simulink model "nonlineardtm"  (R2018b)
settings: configuration reference "Physics" (kept outside this file)
model workspace (MAT data in the model file):
  MCOS : class17 (value not decoded)
undefined symbols (not defined in the file): Aerodynamics, Aligning, Antisway, Brakes, Compliance, ContactPatch, Environment, k1_TireFB_PT1, k1_WheelsFB_PT1, k2_TireFB_PT1, Kinematics, Lateral, Longitudinal, normalizeAngle, omega0_K_Vehicle_radps, omega0_Wheels_radps, Overturning, p_Tires_Pa, Rolling, Scaling, SensorData, Structural, TireSimulation, Turnslip, v0_K_Vehicle_mps, v0z_Wheels_mps, VehicleData, Vertical, Wheels, x0_verticaldynamics, z0_TireDeflection_m
libraries: vehdynlibtire x4, vehdynlibsuspension x2, vrlib x1, vehdynlibeom x1
(part 2 of 5)

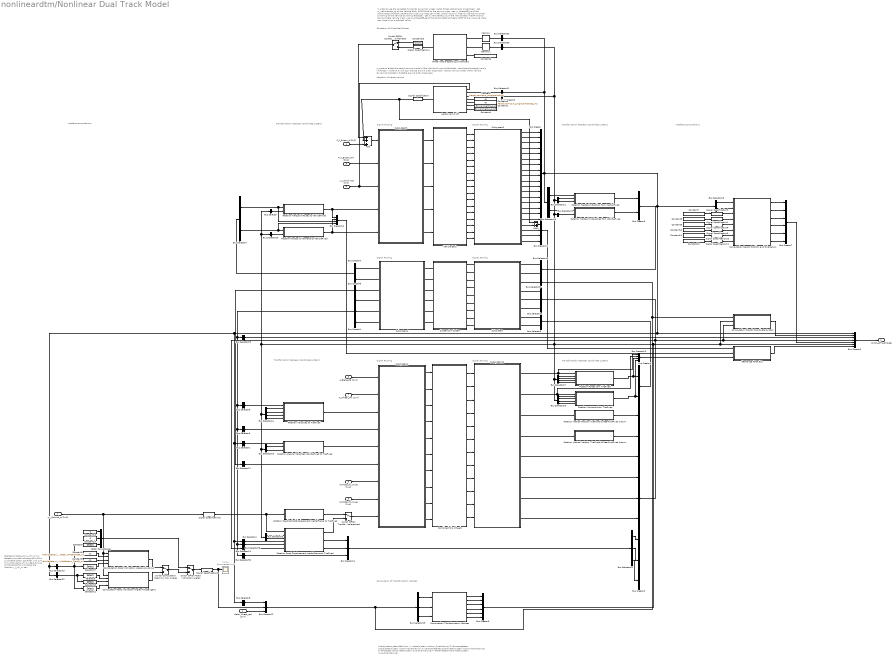
== system nonlineardtm/Nonlinear Dual Track Model ==
  note: Straßenkontaktpunkt  r_I_ITji_m zur Berechnung des Höhhenprofils führt zu algebraischen Schleifen und zum Simulationsabbruch
      | Zur Berechnung ds Höhenprofils wird daher die Position r_I_IAji_m der Anbindungspunkte an die Radaufhängungen verwendet
      | Alternative: Einführung von Verzögerungsgliedern oder Memory-Blöcken
  note: Koordinatensystemdefinition:
      | I: Inertialsystem (z-down Orientierung)
      | F: Fahrzeugfestes Koordinatensystem (z-down-Orientierung)
      | K: Karosseriefestes Koordinatensystem (z-down-Orientierung)
      | R: Radfestes Koordinatensystem (z-up-Orientierung)
      | T: Reifenfestes Koordinatensystem (z-up-Orientierung)
  note: Transformation
      | between coordinate systems
  note: Signal Routing
  note: Signal Routing
  note: Signal Routing
  note: Signal Routing
  note: Transformation
      | between coordinate systems
  note: Signal Routing
  note: Signal Routing
  note: Transformation
      | between coordinate systems
  note: Transformation
      | between coordinate systems
  note: Interface computations
  note: Interface Computations
  note: Computaion of Transformation Matrices
  note: Adaption of Aerodynamics
  note: In order to use the corrected horizontal dynamics wheel inertia forces according to d'Alembert:
      | - set m_VehicleMass_kg of the Vehicle Body 6DOF block to the sprung mass
      | - set m_WheelsFB_kg of the CombinedSlipWheels 2DOF to the unsprung mass per wheel (wheel mass)
      | In order to use the horizontal dynamics of the Vehicle Dynamics Blockset:
      | - set m_VehicleMass_kg of the Vehicle Body 6DOF block to the complete vehicle mass
      | - set m_WheelsFB_kg of the CombinedSlipWheels 2DOF to the unsprung mass per wheel or to a reduced value
  note: In order to adapt the aerodynamics model of the Vehicle Dynamics Blockset:
      | - calculate the aerodynamic lift forces in order to avoid sign change around pitch angle zero. Aerodynamics model of the Vehicle Dynamics blockset is bistable around pitch angle zero.
  note: Correction of d'Alembert Forces
  delta_Wheel_rad [1x4] : Inport
  T_Wheel_Nm [1x4] : Inport  Port=2
  p_Brake_Pa [1x4] : Inport  Port=3
  F_K_Extern_N [3x1] : Inport  Port=4
  T_K_Extern_Nm [3x1] : Inport  Port=5
  v_I_Wind_mps [3x1] : Inport  Port=6
  z_I_Ground_m [1x4] : Inport  Port=7
  lambda_Tji_muex [1x4] : Inport  Port=8
  lambda_Tji_muey [1x4] : Inport  Port=9
  Add : Sum  Inputs=+++
  Add1 : Sum  Inputs=-+
  Aerodynamic Lift : MATLAB Function  TreatAsAtomicUnit=on
  Bus Creator : BusCreator  Inputs=16
  Bus Creator1 : BusCreator  Inputs=3
  Bus Creator10 : BusCreator  Inputs=4
  Bus Creator11 : BusCreator  Inputs=5
  Bus Creator12 : BusCreator  Inputs=3
  Bus Creator13 : BusCreator  Inputs=4
  Bus Creator14 : BusCreator  Inputs=3
  Bus Creator2 : BusCreator  Inputs=9
  Bus Creator3 : BusCreator  Inputs=2
  Bus Creator4 : BusCreator  Inputs=2
  Bus Creator5 : BusCreator  Inputs=7
  Bus Creator6 : BusCreator  Inputs=2
  Bus Creator7 : BusCreator  Inputs=6
  Bus Creator8 : BusCreator  Inputs=1
  Bus Creator9 : BusCreator  Inputs=6
  Bus Selector{,12,20,33} (4 alike) : BusSelector  OutputSignals=A_K_F
  Bus Selector1 : BusSelector  OutputSignals=omega_K_IK_radps
  Bus Selector10 : BusSelector  OutputSignals=phi_IK_rad
  Bus Selector11 : BusSelector  OutputSignals=v_K_IK_mps
  Bus Selector13 : BusSelector  OutputSignals=r_I_IAji_m,v_K_IAji_mps
  Bus Selector14 : BusSelector  OutputSignals=h_ji_m
  Bus Selector15 : BusSelector  OutputSignals=re_ji_m
  Bus Selector16 : BusSelector  OutputSignals=r_F_IAji_m,v_F_IAji_mps
  Bus Selector17 : BusSelector  OutputSignals=F_F_Rji_N
  Bus Selector18 : BusSelector  OutputSignals=r_I_IK_m,A_K_I
  Bus Selector19 : BusSelector  OutputSignals=phi_IK_rad,chi_IO_rad,delta_ji_rad
  Bus Selector2 : BusSelector  OutputSignals=rz_F_Rji_m,re_ji_m,vz_F_Rji_m
  Bus Selector21 : BusSelector  OutputSignals=A_K_I,A_F_I
  Bus Selector22 : BusSelector  OutputSignals=r_I_IAji_m
  Bus Selector23 : BusSelector  OutputSignals=delta_ji_rad
  Bus Selector24 : BusSelector  OutputSignals=A_K_F,A_Rfl_F,A_Rfr_F,A_down_up
  Bus Selector25 : BusSelector  OutputSignals=A_K_F,A_down_up
  Bus Selector26 : BusSelector  OutputSignals=A_K_I,A_F_I
  Bus Selector27 : BusSelector  OutputSignals=A_K_F,A_Rfl_F,A_Rfr_F,A_down_up
  Bus Selector28 : BusSelector  OutputSignals=A_K_F,A_Rfl_F,A_Rfr_F,A_down_up
  Bus Selector29 : BusSelector  OutputSignals=h_ji_m,gamma-tau-nu_rad  OutputAsBus=on
  Bus Selector3 : BusSelector  OutputSignals=F_F_Tji_N,T_F_Tji_Nm
  Bus Selector30 : BusSelector  OutputSignals=v_F_IRji_mps
  Bus Selector31 : BusSelector  OutputSignals=r_I_IRji_m,r_I_ITji_m,v_F_IRji_mps
  Bus Selector32 : BusSelector  OutputSignals=a_K_IK_mps2
  Bus Selector4 : BusSelector  OutputSignals=r_I_IAji_m
  Bus Selector5 : BusSelector  OutputSignals=v_F_IRji_mps
  Bus Selector6 : BusSelector  OutputSignals=gamma-tau-nu_rad
  Bus Selector7 : BusSelector  OutputSignals=F_F_Aji_N,T_F_Aji_Nm
  Bus Selector8 : BusSelector  OutputSignals=phi_IK_rad
  Bus Selector9 : BusSelector  OutputSignals=A_K_I
  Combined Slip Wheels : Subsystem
  Computation Chassis Coordinate System : Subsystem
  Computation Road Inclination Angles Arkussinus : MATLAB Function  TreatAsAtomicUnit=on
  Computation Road Inclination Angles Arkustangens : MATLAB Function  TreatAsAtomicUnit=on
  Computation Sensor Position and Orientation : MATLAB Function  TreatAsAtomicUnit=on
  Computation Transformation Matrices : MATLAB Function  TreatAsAtomicUnit=on
  Constant : Constant  Value=Aerodynamics.cl_LongitudinalLift
  Constant1 : Constant  Value=Environment.t_Air_K
  Constant10 : Constant  Value=SensorData.phi0_K_KS1_rad
  Constant11 : Constant  Value=SensorData.phi0_K_KS2_rad
  Constant12 : Constant  Value=SensorData.phi0_K_KS3_rad
  Constant13 : Constant  Value=0
  Constant14 : Constant  Value=0
  Constant15 : Constant  Value=[0;0;0]
  Constant2 : Constant  Value=[VehicleData.l_WheelbaseF_m VehicleData.l_WheelbaseR_m]
  Constant3 : Constant  Value=Aerodynamics.A_LongitudinalDrag_m2
  Constant4 : Constant  Value=Environment.p_Air_Pa
  Constant5 : Constant  Value=[VehicleData.w_TrackF_m VehicleData.w_TrackR_m]
  Constant6 : Constant  Value=Wheels.m_WheelsFB_kg
  Constant7 : Constant  Value=SensorData.r_K_KS1_m
  Constant8 : Constant  Value=SensorData.r_K_KS2_m
  Constant9 : Constant  Value=SensorData.r_K_KS3_m
  Memory : Memory
  Memory1 : Memory
  Rearrange Force Bus : Subsystem
  Rotation Angular Velocities VehicleFixed to TireFixed : MATLAB Function  TreatAsAtomicUnit=on
  Rotation Forces from TireFixed : MATLAB Function  TreatAsAtomicUnit=on
  Rotation Hardpoint Forces to VehicleFixed : MATLAB Function  TreatAsAtomicUnit=on
  Rotation Hardpoint Moments to VehicleFixed : MATLAB Function  TreatAsAtomicUnit=on
  Rotation Hardpoint Position from InertialFixed : MATLAB Function  TreatAsAtomicUnit=on
  Rotation Hardpoint Velocities from VehicleFixed : MATLAB Function  TreatAsAtomicUnit=on
  Rotation Moments from TireFixed : MATLAB Function  TreatAsAtomicUnit=on
  Rotation Road Displacement InertialFrame to TireFixed : MATLAB Function  TreatAsAtomicUnit=on
  Rotation RoadVerticalDisplacement InertialFrame to TireFixed : Subsystem
  Rotation Velocities to TireFixed : MATLAB Function  TreatAsAtomicUnit=on
  Rotation Vertical Position TireFixed to RearAxleFixed z-down : Subsystem
  Rotation Vertical Velocity TireFixed to RearAxleFixed z-down : Subsystem
  Scope : Scope  Commented=on
  Selector20 : Selector  NumberOfDimensions=2  InputPortWidth=3  IndexOptions=Index vector (dialog),Select all  Indices=2,1  OutputSizes=1,1
  Selector21 : Selector  InputPortWidth=3  IndexOptions=Index vector (dialog)  Indices=3  OutputSizes=1
  Selector3 : Selector  InputPortWidth=3  IndexOptions=Index vector (dialog)  Indices=3  OutputSizes=1
  Selector37 : Selector  InputPortWidth=3  IndexOptions=Index vector (dialog)  Indices=3  OutputSizes=1
  Selector6 : Selector  NumberOfDimensions=2  InputPortWidth=3  IndexOptions=Index vector (dialog),Select all  Indices=1,1  OutputSizes=1,1
  Signal Specification{,1..4,8..11} (9 alike) : SignalSpecification  Dimensions=[3,1]
  Signal Specification5 : SignalSpecification  Dimensions=[1,4]
  Subsystem : Subsystem
  Subsystem1 : Subsystem
  Subsystem11 : Subsystem
  Subsystem2 : Subsystem
  Subsystem3 : Subsystem
  Subsystem4 : Subsystem
  Suspension System : Subsystem
  Switch Computation Road Inclination Angles : ManualSwitch
  Switch Off/On Correction Horizontal Dynamics Wheel Inertia according d'Alembert : ManualSwitch
  Switch Off/On Road Inclination Angles : ManualSwitch
  Switch Off/On Transformation Ground Displacement : ManualSwitch
  Vector Concatenate : Concatenate  NumInputs=3
  Vehicle Body : Subsystem
  Wheel Inertia according d'Alembert : MATLAB Function  TreatAsAtomicUnit=on
  SimDualTrackModel : Outport
  wires:
  Subsystem2/15(v_K_IAji_mps [3x4]) -> Bus Creator/15  "v_K_IAji_mps"
  Subsystem2/14(r_K_KAji_m [3x4]) -> Bus Creator/14  "r_K_KAji_m"
  Subsystem4/5(gamma-tau-nu_rad) -> Bus Creator1/2  "gamma-tau-nu_rad"
  Subsystem2/10(omega_K_IK_radps [3x1]) -> Bus Creator/10  "omega_K_IK_radps"
  Subsystem2/4(phi_IK_rad [3x1]) -> Bus Creator/4  "phi_IK_rad"
  v_I_Wind_mps [3x1]/1 -> Subsystem3/3(v_I_Wind_mps), Aerodynamic Lift/1(v_I_Wind_mps)  "v_I_Wind_mps"
  T_K_Extern_Nm [3x1]/1 -> Subsystem3/2(T_K_Extern_Nm)  "T_K_Ext_Nm"
  Add/1 -> Subsystem3/1(F_K_Extern_N)  "F_K_Ext_N"
  Subsystem11/6(omegay_Rji_Rji_radps) -> Bus Creator2/4  "omegay_Rji_Rji_radps"
  Subsystem11/4(vz_Tji_Rji_mps) -> Rotation Vertical Velocity TireFixed to RearAxleFixed z-down/1(vz_Tji_Rji_mps)  "vz_Tji_Rji_mps"
  Bus Creator2/1 -> Bus Selector15/1, Bus Selector2/1, Bus Creator5/4, Computation Chassis Coordinate System/3(Wheel)  "SimWheel"
  Bus Selector2/1 -> Subsystem/4(rz_F_IRji_m)  "<rz_F_Rji_m>"
  Bus Selector2/2 -> Subsystem/5(re_Rji_m)  "<re_ji_m>"
  Bus Selector2/3 -> Subsystem/6(vz_F_IRji_mps)  "<vz_F_Rji_m>"
  Bus Creator3/1 -> Bus Selector3/1
  Bus Selector3/1 -> Subsystem/7(F_F_Tji_N)  "<F_F_Tji_N>"
  Bus Selector3/2 -> Subsystem/8(T_F_Tji_Nm)  "<T_F_Tji_Nm>"
  z_I_Ground_m [1x4]/1 -> Signal Specification5/1, Computation Road Inclination Angles Arkustangens/1(z_I_Ground_m), Computation Road Inclination Angles Arkussinus/1(z_I_Ground_m)
  Subsystem2/1(r_I_IK_m [3x1]) -> Bus Creator/1  "r_I_IK_m"
  Subsystem2/2(v_I_IK_mps [3x1]) -> Bus Creator/2  "v_I_IK_mps"
  Subsystem2/13(v_I_IAji_mps [3x4]) -> Bus Creator/13  "v_I_IAji_mps"
  Subsystem2/7(v_K_IK_mps [3x1]) -> Bus Creator/7  "v_K_IK_mps"
  Subsystem2/8(a_K_IK_mps2 [3x1]) -> Bus Creator/8  "a_K_IK_mps2"
  Bus Selector8/1 -> Bus Creator12/1  "<phi_IK_rad>"
  Bus Selector1/1 -> Rotation Angular Velocities VehicleFixed to TireFixed/1(omega_K_IK_radps)  "<omega_K_IK_radps>"
  Bus Selector6/1 -> Subsystem1/4(gamma-tau-nu_rad)  "<gamma-tau-nu_rad>"
  Bus Creator4/1 -> Bus Selector7/1
  Bus Creator5/1 -> SimDualTrackModel/1
  Bus Creator1/1 -> Bus Selector30/1, Bus Selector14/1, Bus Selector6/1, Bus Selector5/1, Bus Selector29/1
  Subsystem2/16(A_K_I [3x3]) -> Bus Creator/16  "A_K_I"
  Subsystem2/12(r_I_IAji_m [3x4]) -> Bus Creator/12  "r_I_IAji_m"
  Subsystem11/5(re_ji_m) -> Bus Creator2/3  "re_ji_m"
  Bus Selector7/1 -> Bus Creator10/3, Rotation Hardpoint Forces to VehicleFixed/1(F_F_Aji_N)  "<F_F_Aji_N>"
  Bus Selector7/2 -> Bus Creator10/4, Rotation Hardpoint Moments to VehicleFixed/1(T_F_Aji_Nm)  "<T_F_Aji_Nm>"
  Rotation Hardpoint Position from InertialFixed/1(r_F_IAji_m) -> Bus Creator6/1  "r_F_IAji_m"
  Rotation Hardpoint Forces to VehicleFixed/1(F_K_Aji_N) -> Bus Creator10/1, Subsystem3/4(F_K_Aji_N)  "F_K_Aji_N"
  Rotation Hardpoint Moments to VehicleFixed/1(T_K_Aji_Nm) -> Bus Creator10/2, Subsystem3/5(T_K_Aji_Nm)  "T_K_Aji_Nm"
  Bus Selector5/1 -> Rotation Velocities to TireFixed/1(v_F_IRji_mps)  "<v_F_IRji_mps>"
  Rotation Velocities to TireFixed/1(v_Tji_Rji_mps) -> Subsystem1/3(v_Tji_Rji_mps)  "v_Tji_Rji_mps"
  Bus Selector10/1 -> Selector21/1, Selector37/1, Selector3/1  "<phi_IK_rad>"
  Constant2/1 -> Computation Road Inclination Angles Arkussinus/2(l_WheelbaseFB_m)
  Constant5/1 -> Computation Road Inclination Angles Arkussinus/3(w_TrackFB_m)
  Bus Selector13/2 -> Rotation Hardpoint Velocities from VehicleFixed/1(v_K_IAji_mps)  "<v_K_IAji_mps>"
  Signal Specification2/1 -> Bus Creator12/2, Scope/1  "chi_IO_rad"
  Bus Selector13/1 -> Rotation Hardpoint Position from InertialFixed/1(r_I_IAji_m)  "<r_I_IAji_m>"
  Bus Selector4/1 -> Rotation Road Displacement InertialFrame to TireFixed/4(r_I_IAji_m)  "<r_I_IAji_m>"
  Bus Selector14/1 -> Rotation Road Displacement InertialFrame to TireFixed/5(h_ji_m)  "<h_ji_m>"
  Bus Selector15/1 -> Rotation Road Displacement InertialFrame to TireFixed/6(re_ji_m)  "<re_ji_m>"
  Bus Selector16/1 -> Subsystem/1(r_F_IAji_m)  "<r_F_IAji_m>"
  Bus Selector16/2 -> Subsystem/2(v_F_IAji_mps)  "<v_F_IAji_mps>"
  Bus Creator6/1 -> Bus Selector16/1
  Subsystem11/7(kappa_ji) -> Bus Creator2/5  "kappa_ji"
  Subsystem11/8(alpha_ji_rad) -> Bus Creator2/6  "alpha_ji_rad"
  Rotation Road Displacement InertialFrame to TireFixed/3(r_I_ITji_m) -> Bus Creator14/2  "r_I_ITji_m"
  Bus Selector18/2 -> Computation Sensor Position and Orientation/2(A_K_I)  "<A_K_I>"
  Computation Sensor Position and Orientation/6(A_S3_I) -> Bus Creator7/6  "A_S3_I"
  Computation Sensor Position and Orientation/1(r_I_IS1_m) -> Bus Creator7/1  "r_I_IS1_m"
  Computation Sensor Position and Orientation/2(r_I_IS2_m) -> Bus Creator7/2  "r_I_IS2_m"
  Computation Sensor Position and Orientation/3(r_I_IS3_m) -> Bus Creator7/3  "r_I_IS3_m"
  Computation Sensor Position and Orientation/4(A_S1_I) -> Bus Creator7/4  "A_S1_I"
  Computation Sensor Position and Orientation/5(A_S2_I) -> Bus Creator7/5  "A_S2_I"
  Bus Creator7/1 -> Bus Creator5/5  "SimSensor"
  Bus Selector18/1 -> Computation Sensor Position and Orientation/1(r_I_IK_m)  "<r_I_IK_m>"
  Constant7/1 -> Signal Specification3/1
  Constant8/1 -> Signal Specification1/1
  Constant9/1 -> Signal Specification8/1
  Constant10/1 -> Signal Specification9/1
  Constant11/1 -> Signal Specification10/1
  Constant12/1 -> Signal Specification11/1
  Subsystem11/1(F_Tji_Tji_N) -> Rotation Forces from TireFixed/1(F_Tji_Tji_N), Bus Creator13/1  "F_Tji_Tji_N"
  Rotation Hardpoint Velocities from VehicleFixed/1(v_F_IAji_mps) -> Bus Creator6/2  "v_F_IAji_mps"
  Rotation Angular Velocities VehicleFixed to TireFixed/1(omega_Tji_ITji_radps) -> Subsystem1/5(omega_Tji_ITji_radps)  "omega_Tji_ITji_radps"
  Signal Specification5/1 -> Rotation RoadVerticalDisplacement InertialFrame to TireFixed/1(z_I_Ground_m), Rotation Road Displacement InertialFrame to TireFixed/1(z_I_Ground_m)
  Subsystem4/3(F_F_Rji_N) -> Bus Creator8/1  "F_F_Rji_N"
  delta_Wheel_rad [1x4]/1 -> Bus Creator12/3  "delta_ji_rad"
  Rotation Forces from TireFixed/1(F_F_Tji_N) -> Bus Creator13/3, Bus Creator3/1  "F_F_Tji_N"
  Rotation Moments from TireFixed/1(T_F_Tji_Nm) -> Bus Creator13/4, Bus Creator3/2  "T_F_Tji_Nm"
  Rotation Vertical Position TireFixed to RearAxleFixed z-down/1(rz_F_Rji_m) -> Bus Creator2/1  "rz_F_Rji_m"
  Rotation Vertical Velocity TireFixed to RearAxleFixed z-down/1(vz_F_Rji_mps) -> Bus Creator2/2  "vz_F_Rji_m"
  Subsystem/1(VehP [3x4]) -> Suspension System/1(VehP [3x4])
  Subsystem/2(VehV [3x4]) -> Suspension System/2(VehV [3x4])
  Subsystem/3(StrgAngF [1x2]) -> Suspension System/3(StrgAngF [1x2])
  Subsystem/4(WhlPz [1x4]) -> Suspension System/4(WhlPz [1x4])
  Subsystem/5(WhlRe [1x4]) -> Suspension System/5(WhlRe [1x4])
  Subsystem/6(WhlVz [1x4]) -> Suspension System/6(WhlVz [1x4])
  Subsystem/7(WhlFx [1x4]) -> Suspension System/7(WhlFx [1x4])
  Subsystem/8(WhlFy [1x4]) -> Suspension System/8(WhlFy [1x4])
  Subsystem/9(WhlM [3x4]) -> Suspension System/9(WhlM [3x4])
  Suspension System/1(VehF [3x4]) -> Subsystem4/1(VehF [3x4])
  Suspension System/2(VehM [3x4]) -> Subsystem4/2(VehM [3x4])
  Suspension System/3(WhlF [3x4]) -> Subsystem4/3(WhlF [3x4])
  Suspension System/4(WhlV [3x4]) -> Subsystem4/4(WhlV [3x4])
  Suspension System/5(WhlAng [3x4]) -> Subsystem4/5(WhlAng [3x4])
  Suspension System/6(SuspH [1x4]) -> Subsystem4/6(SuspH [1x4])
  Subsystem4/1(F_F_Aji_N) -> Bus Creator4/1  "F_F_Aji_N"
  Subsystem4/2(T_F_Aji_Nm) -> Bus Creator4/2  "T_F_Aji_Nm"
  Subsystem4/6(h_ji_m) -> Bus Creator1/3  "h_ji_m"
  Subsystem4/4(v_F_IRji_mps) -> Bus Creator1/1  "v_F_IRji_mps"
  Constant13/1 -> Vector Concatenate/1
  Constant14/1 -> Vector Concatenate/2
  Selector3/1 -> Vector Concatenate/3
  Selector37/1 -> Computation Road Inclination Angles Arkussinus/4(phiz_IK_rad)
  Vector Concatenate/1 -> Switch Off/On Road Inclination Angles/1
  Selector6/1 -> Computation Road Inclination Angles Arkustangens/2(rx_I_IAji_m)
  Selector20/1 -> Computation Road Inclination Angles Arkustangens/3(ry_I_IAji_m)
  Selector21/1 -> Computation Road Inclination Angles Arkustangens/4(phiz_IK_rad)
  Computation Road Inclination Angles Arkussinus/1(chi) -> Switch Computation Road Inclination Angles/1
  Computation Road Inclination Angles Arkustangens/1(chi) -> Switch Computation Road Inclination Angles/2
  Signal Specification3/1 -> Computation Sensor Position and Orientation/3(r_K_KS1_m)
  Signal Specification1/1 -> Computation Sensor Position and Orientation/4(r_K_KS2_m)
  Signal Specification8/1 -> Computation Sensor Position and Orientation/5(r_K_KS3_m)
  Signal Specification9/1 -> Computation Sensor Position and Orientation/6(phi0_K_KS1_rad)
  Signal Specification10/1 -> Computation Sensor Position and Orientation/7(phi0_K_KS2_rad)
  Signal Specification11/1 -> Computation Sensor Position and Orientation/8(phi0_K_KS3_rad)
  Subsystem2/9(vdot_K_IK_mps2 [3x1]) -> Bus Creator/9  "vdot_K_IK_mps2"
  Subsystem3/5(MSusp [3x4]) -> Vehicle Body/5(MSusp [3x4])
  Combined Slip Wheels/1(Fx [1x4]) -> Subsystem11/1(Fx [1x4])
  Combined Slip Wheels/2(Fy [1x4]) -> Subsystem11/2(Fy [1x4])
  Combined Slip Wheels/3(Fz [1x4]) -> Subsystem11/3(Fz [1x4])
  Combined Slip Wheels/5(My [1x4]) -> Subsystem11/5(My [1x4])
  Combined Slip Wheels/6(Mz [1x4]) -> Subsystem11/6(Mz [1x4])
  Combined Slip Wheels/7(z [1x4]) -> Subsystem11/7(z [1x4])
  Combined Slip Wheels/8(zdot [1x4]) -> Subsystem11/8(zdot [1x4])
  Combined Slip Wheels/9(Re [1x4]) -> Subsystem11/9(Re [1x4])
  Combined Slip Wheels/10(omega [1x4]) -> Subsystem11/10(omega [1x4])
  Combined Slip Wheels/11(Kappa [1x4]) -> Subsystem11/11(Kappa [1x4])
  Subsystem11/2(T_Tji_Tji_Nm) -> Rotation Moments from TireFixed/1(T_Tji_Tji_Nm), Bus Creator13/2  "T_Tji_Tji_Nm"
  Subsystem11/3(rz_Tji_Rji_m) -> Rotation Vertical Position TireFixed to RearAxleFixed z-down/1(rz_Tji_Rji_m)  "rz_Tji_Rji_m"
  p_Brake_Pa [1x4]/1 -> Subsystem1/1(p_Brake_Pa)
  T_Wheel_Nm [1x4]/1 -> Subsystem1/2(T_Wheel_Nm)
  lambda_Tji_muex [1x4]/1 -> Subsystem1/7(lambda_Tji_muex [1x4])
  lambda_Tji_muey [1x4]/1 -> Subsystem1/8(lambda_Tji_muey [1x4])
  Switch Off/On Transformation Ground Displacement/1 -> Subsystem1/9(z_Tji_Ground_m [1x4])
  Rotation RoadVerticalDisplacement InertialFrame to TireFixed/1(z_Tji_Ground_m) -> Switch Off/On Transformation Ground Displacement/1  "z_Tji_Ground_m"
  Rotation Road Displacement InertialFrame to TireFixed/1(z_Tji_Ground_m) -> Switch Off/On Transformation Ground Displacement/2  "z_Tji_Ground_m"
  Bus Creator8/1 -> Bus Selector17/1
  Bus Selector17/1 -> Subsystem1/6(F_F_Rji_N [3x4])  "<F_F_Rji_N>"
  Switch Computation Road Inclination Angles/1 -> Switch Off/On Road Inclination Angles/2
  Switch Off/On Road Inclination Angles/1 -> Signal Specification2/1
  Subsystem1/1(BrkPrs [1x4]) -> Combined Slip Wheels/1(BrkPrs [1x4])
  Subsystem1/2(AxlTrq [1x4]) -> Combined Slip Wheels/2(AxlTrq [1x4])
  Subsystem1/3(Vx [1x4]) -> Combined Slip Wheels/3(Vx [1x4])
  Subsystem1/4(Vy [1x4]) -> Combined Slip Wheels/4(Vy [1x4])
  Subsystem1/5(Camber [1x4]) -> Combined Slip Wheels/5(Camber [1x4])
  Subsystem1/6(YawRate [1x4]) -> Combined Slip Wheels/6(YawRate [1x4])
  Subsystem1/7(Prs [1x4]) -> Combined Slip Wheels/7(Prs [1x4])
  Subsystem1/8(Gnd [1x4]) -> Combined Slip Wheels/8(Gnd [1x4])
  Subsystem1/9(Fext [1x4]) -> Combined Slip Wheels/9(Fext [1x4])
  Subsystem1/10(ScaleFctrs [27x4]) -> Combined Slip Wheels/10(ScaleFctrs [27x4])
  Combined Slip Wheels/12(Alpha [1x4]) -> Subsystem11/12(Alpha [1x4])
  Computation Transformation Matrices/1(A_K_I) -> Bus Creator9/1  "A_K_I"
  Computation Transformation Matrices/2(A_K_F) -> Bus Creator9/2  "A_K_F"
  Computation Transformation Matrices/3(A_F_I) -> Bus Creator9/3  "A_F_I"
  Computation Transformation Matrices/4(A_Rfl_F) -> Bus Creator9/4  "A_Rfl_F"
  Computation Transformation Matrices/5(A_Rfr_F) -> Bus Creator9/5  "A_Rfr_F"
  Computation Transformation Matrices/6(A_down_up) -> Bus Creator9/6  "A_down_up"
  Bus Selector/1 -> Rotation Hardpoint Forces to VehicleFixed/2(A_K_F)  "<A_K_F>"
  Bus Selector20/1 -> Rotation Hardpoint Moments to VehicleFixed/2(A_K_F)  "<A_K_F>"
  Bus Selector12/1 -> Rotation Hardpoint Velocities from VehicleFixed/2(A_K_F)  "<A_K_F>"
  Bus Selector21/1 -> Rotation Hardpoint Position from InertialFixed/2(A_K_I)  "<A_K_I>"
  Bus Selector21/2 -> Rotation Hardpoint Position from InertialFixed/3(A_F_I)  "<A_F_I>"
  Bus Selector24/1 -> Rotation Velocities to TireFixed/2(A_K_F)  "<A_K_F>"
  Bus Selector24/2 -> Rotation Velocities to TireFixed/3(A_Rfl_F)  "<A_Rfl_F>"
  Bus Selector24/3 -> Rotation Velocities to TireFixed/4(A_Rfr_F)  "<A_Rfr_F>"
  Bus Selector24/4 -> Rotation Velocities to TireFixed/5(A_down_up)  "<A_down_up>"
  Bus Selector25/1 -> Rotation Angular Velocities VehicleFixed to TireFixed/2(A_K_F)  "<A_K_F>"
  Bus Selector25/2 -> Rotation Angular Velocities VehicleFixed to TireFixed/3(A_down_up)  "<A_down_up>"
  Bus Selector26/1 -> Rotation Road Displacement InertialFrame to TireFixed/2(A_K_I)  "<A_K_I>"
  Bus Selector26/2 -> Rotation Road Displacement InertialFrame to TireFixed/3(A_F_I)  "<A_F_I>"
  Bus Selector27/1 -> Rotation Forces from TireFixed/2(A_K_F)  "<A_K_F>"
  Bus Selector27/2 -> Rotation Forces from TireFixed/3(A_Rfl_F)  "<A_Rfl_F>"
  Bus Selector27/3 -> Rotation Forces from TireFixed/4(A_Rfr_F)  "<A_Rfr_F>"
  Bus Selector27/4 -> Rotation Forces from TireFixed/5(A_down_up)  "<A_down_up>"
  Bus Selector28/1 -> Rotation Moments from TireFixed/2(A_K_F)  "<A_K_F>"
  Bus Selector28/2 -> Rotation Moments from TireFixed/3(A_Rfl_F)  "<A_Rfl_F>"
  Bus Selector28/3 -> Rotation Moments from TireFixed/4(A_Rfr_F)  "<A_Rfr_F>"
  Bus Selector28/4 -> Rotation Moments from TireFixed/5(A_down_up)  "<A_down_up>"
  Bus Selector22/1 -> Selector20/1, Selector6/1  "<r_I_IAji_m>"
  Subsystem2/17(F_K_g_N [3x1]) -> Bus Creator11/1  "F_K_g_N"
  Add1/1 -> Bus Creator11/2  "F_K_d_N"
  Subsystem2/19(T_K_d_Nm [3x1]) -> Bus Creator11/3  "T_K_d_Nm"
  Subsystem2/20(F_K_sum_N [3x1]) -> Bus Creator11/4  "F_K_sum_N"
  Subsystem2/21(T_K_sum_Nm [3x1]) -> Bus Creator11/5  "T_K_sum_Nm"
  Subsystem3/4(FSusp [3x4]) -> Vehicle Body/4(FSusp [3x4])
  Vehicle Body/1(InertFrm.Cg.Disp [3x1]) -> Subsystem2/1(InertFrm.Cg.Disp [3x1])
  Vehicle Body/2(InertFrm.Cg.Vel [3x1]) -> Subsystem2/2(InertFrm.Cg.Vel [3x1])
  Vehicle Body/3(InertFrm.Cg.Ang [3x1]) -> Subsystem2/3(InertFrm.Cg.Ang [3x1])
  Vehicle Body/4(InertFrm.Axl.Disp [3x4]) -> Subsystem2/4(InertFrm.Axl.Disp [3x4])
  Vehicle Body/5(InertFrm.Axl.Vel [3x4]) -> Subsystem2/5(InertFrm.Axl.Vel [3x4])
  Vehicle Body/6(BdyFrm.Cg.Vel [3x1]) -> Subsystem2/6(BdyFrm.Cg.Vel [3x1])
  Vehicle Body/7(BdyFrm.Cg.AngVel [3x1]) -> Subsystem2/7(BdyFrm.Cg.AngVel [3x1])
  Vehicle Body/8(BdyFrm.Cg.Acc [3x1]) -> Subsystem2/8(BdyFrm.Cg.Acc [3x1])
  Vehicle Body/9(BdyFrm.Cg.AccRel [3x1]) -> Subsystem2/9(BdyFrm.Cg.AccRel [3x1])
  Vehicle Body/10(BdyFrm.Axl.Disp [3x4]) -> Subsystem2/10(BdyFrm.Axl.Disp [3x4])
  Vehicle Body/11(BdyFrm.Axl.Vel [3x4]) -> Subsystem2/11(BdyFrm.Axl.Vel [3x4])
  Vehicle Body/12(BdyFrm.Cg.DCM [3x3]) -> Subsystem2/12(BdyFrm.Cg.DCM [3x3])
  Vehicle Body/13(BdyFrm.Forces.Grvty [3x1]) -> Subsystem2/13(BdyFrm.Forces.Grvty [3x1])
  Vehicle Body/14(BdyFrm.Forces.Drag [3x1]) -> Subsystem2/14(BdyFrm.Forces.Drag [3x1])
  Vehicle Body/15(BdyFrm.Moments.Drag [3x1]) -> Subsystem2/15(BdyFrm.Moments.Drag [3x1])
  Vehicle Body/16(BdyFrm.Forces.Body [3x1]) -> Subsystem2/16(BdyFrm.Forces.Body [3x1])
  Vehicle Body/17(BdyFrm.Moments.Body [3x1]) -> Subsystem2/17(BdyFrm.Moments.Body [3x1])
  Subsystem2/11(alpha_K_IK_radps2 [3x1]) -> Bus Creator/11  "alpha_K_IK_radps2"
  Subsystem2/3(a_I_IK_mps2 [3x1]) -> Bus Creator/3  "a_I_IK_mps2"
  Subsystem2/5(omega_I_IK_radps [3x1]) -> Bus Creator/5  "omega_I_IK_radps"
  Subsystem2/6(alpha_I_IK_radps2 [3x1]) -> Bus Creator/6  "alpha_I_IK_radps2"
  Bus Creator11/1 -> Rearrange Force Bus/1(VehicleForces)  "VehicleForces"
  Bus Creator10/1 -> Rearrange Force Bus/2(SuspensionForces)  "SuspensionForces"
  Bus Creator13/1 -> Rearrange Force Bus/3(TireForces)  "TireForces"
  Rearrange Force Bus/1(Force) -> Bus Creator5/7  "SimForce"
  Rotation Road Displacement InertialFrame to TireFixed/2(r_I_IRji_m) -> Bus Creator14/1  "r_I_IRji_m"
  Subsystem3/1(FExt [3x1]) -> Vehicle Body/1(FExt [3x1])
  Subsystem3/2(MExt [3x1]) -> Vehicle Body/2(MExt [3x1])
  Subsystem3/3(WindXYZ [3x1]) -> Vehicle Body/3(WindXYZ [3x1])
  Bus Creator12/1 -> Bus Selector23/1, Computation Chassis Coordinate System/1(TransformationAngles), Bus Selector19/1  "TransformationAngles"
  Bus Selector19/1 -> Computation Transformation Matrices/1(phi)  "<phi_IK_rad>"
  Bus Selector19/2 -> Computation Transformation Matrices/2(chi)  "<chi_IO_rad>"
  Bus Selector19/3 -> Computation Transformation Matrices/3(delta)  "<delta_ji_rad>"
  Bus Selector23/1 -> Subsystem/3(delta_ji_rad)  "<delta_ji_rad>"
  Computation Chassis Coordinate System/1(Chassis) -> Bus Creator5/2  "SimChassis"
  Bus Selector29/1 -> Bus Creator5/3  "SimSuspension"
  Bus Selector30/1 -> Bus Creator14/3  "<v_F_IRji_mps>"
  Bus Creator14/1 -> Bus Selector31/1
  Bus Selector31/2 -> Bus Creator2/8  "<r_I_ITji_m>"
  Bus Selector31/3 -> Bus Creator2/9  "<v_F_IRji_mps>"
  Bus Selector31/1 -> Bus Creator2/7  "<r_I_IRji_m>"
  Combined Slip Wheels/4(Mx [1x4]) -> Subsystem11/4(Mx [1x4])
  Aerodynamic Lift/1(F_K_Lift_N) -> Signal Specification/1
  F_K_Extern_N [3x1]/1 -> Add/3
  Bus Selector9/1 -> Aerodynamic Lift/3(A_K_I)  "<A_K_I>"
  Constant/1 -> Aerodynamic Lift/4(cl_LongitudinalLift)
  Constant1/1 -> Aerodynamic Lift/6(t_Air_K)
  Bus Selector11/1 -> Aerodynamic Lift/2(v_K_IK_mps)  "<v_K_IK_mps>"
  Constant3/1 -> Aerodynamic Lift/5(A_LongitudinalDrag_m2)
  Constant4/1 -> Aerodynamic Lift/7(p_Air_Pa)
  Signal Specification/1 -> Add/2, Add1/1
  Subsystem2/18(F_K_d_N [3x1]) -> Add1/2  "F_K_d_N"
  Switch Off/On Correction Horizontal Dynamics Wheel Inertia according d'Alembert/1 -> Add/1
  Constant6/1 -> Wheel Inertia according d'Alembert/3(m_WheelsFB_kg)
  Bus Selector32/1 -> Memory/1  "<a_K_IK_mps2>"
  Signal Specification4/1 -> Switch Off/On Correction Horizontal Dynamics Wheel Inertia according d'Alembert/2
  Bus Selector33/1 -> Memory1/1  "<A_K_F>"
  Constant15/1 -> Switch Off/On Correction Horizontal Dynamics Wheel Inertia according d'Alembert/1
  Memory/1 -> Wheel Inertia according d'Alembert/1(a_K_IK_mps2)
  Bus Creator9/1 -> Bus Selector28/1, Bus Selector27/1, Bus Selector24/1, Bus Selector26/1, Bus Selector25/1, Bus Selector20/1, Bus Selector/1, Bus Selector33/1, Bus Selector9/1, Bus Selector21/1, Bus Selector12/1, Bus Creator5/6, Computation Chassis Coordinate System/2(Transformation)
  Wheel Inertia according d'Alembert/1(F_K_dAlembert_N) -> Signal Specification4/1
  Bus Creator/1 -> Bus Selector32/1, Bus Selector11/1, Bus Selector13/1, Bus Selector8/1, Bus Selector4/1, Bus Selector1/1, Bus Selector10/1, Bus Selector22/1, Bus Creator5/1, Bus Selector18/1
  Memory1/1 -> Wheel Inertia according d'Alembert/2(A_K_F)

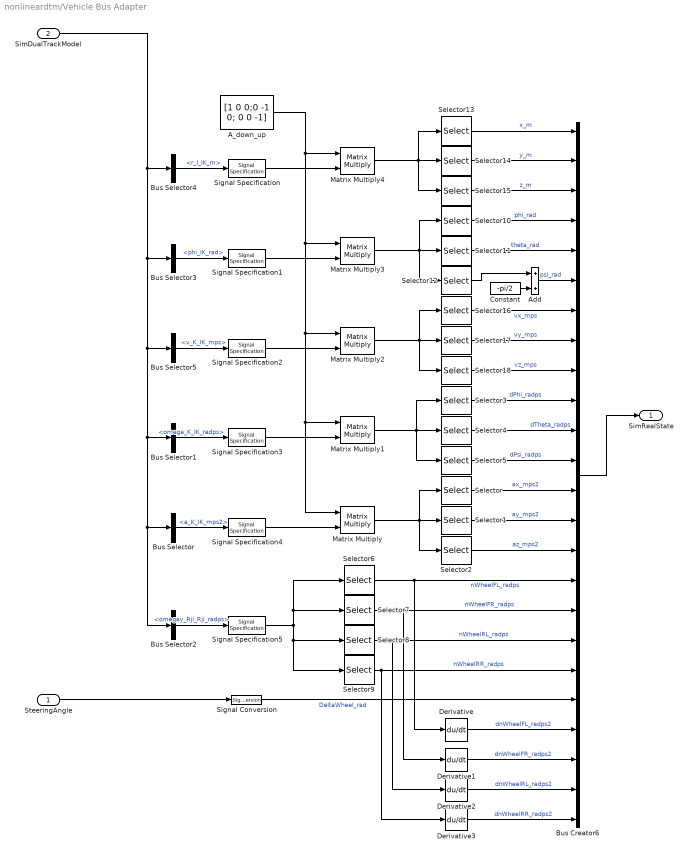
== system nonlineardtm/Vehicle Bus Adapter ==
  SteeringAngle : Inport
  SimDualTrackModel : Inport  Port=2
  A_down_up : Constant  Value=[1 0 0;0 -1 0; 0 0 -1]
  Add : Sum
  Bus Creator6 : BusCreator  Inputs=24
  Bus Selector : BusSelector  OutputSignals=signal1.a_K_IK_mps2
  Bus Selector1 : BusSelector  OutputSignals=signal1.omega_K_IK_radps
  Bus Selector2 : BusSelector  OutputSignals=SimWheel.omegay_Rji_Rji_radps
  Bus Selector3 : BusSelector  OutputSignals=signal1.phi_IK_rad
  Bus Selector4 : BusSelector  OutputSignals=signal1.r_I_IK_m
  Bus Selector5 : BusSelector  OutputSignals=signal1.v_K_IK_mps
  Constant : Constant  Value=-pi/2
  Derivative{,1..3} (4 alike) : Derivative
  Matrix Multiply{,1..4} (5 alike) : Product  Multiplication=Matrix(*)
  Selector{,3,10,13,16} (5 alike) : Selector  InputPortWidth=3  IndexOptions=Index vector (dialog)  Indices=[1]  OutputSizes=1
  Selector{1,4,11,14,17} (5 alike) : Selector  InputPortWidth=3  IndexOptions=Index vector (dialog)  Indices=[2]  OutputSizes=1
  Selector{2,5,12,15,18} (5 alike) : Selector  InputPortWidth=3  IndexOptions=Index vector (dialog)  Indices=[3]  OutputSizes=1
  Selector6 : Selector  InputPortWidth=4  IndexOptions=Index vector (dialog)  Indices=[1]  OutputSizes=1
  Selector7 : Selector  InputPortWidth=4  IndexOptions=Index vector (dialog)  Indices=[2]  OutputSizes=1
  Selector8 : Selector  InputPortWidth=4  IndexOptions=Index vector (dialog)  Indices=[3]  OutputSizes=1
  Selector9 : Selector  InputPortWidth=4  IndexOptions=Index vector (dialog)  Indices=4  OutputSizes=1
  Signal Conversion : SignalConversion  OverrideOpt=off
  Signal Specification{,1..4} (5 alike) : SignalSpecification  Dimensions=[3,1]
  Signal Specification5 : SignalSpecification  Dimensions=[1,4]
  SimRealState : Outport
  wires:
  Bus Selector4/1 -> Signal Specification/1  "<r_I_IK_m>"
  Matrix Multiply2/1 -> Selector18/1, Selector16/1, Selector17/1
  Selector14/1 -> Bus Creator6/2  "y_m"
  Matrix Multiply/1 -> Selector2/1, Selector/1, Selector1/1
  Selector1/1 -> Bus Creator6/14  "ay_mps2"
  Bus Selector2/1 -> Signal Specification5/1  "<omegay_Rji_Rji_radps>"
  Selector16/1 -> Bus Creator6/7  "vx_mps"
  Selector17/1 -> Bus Creator6/8  "vy_mps"
  Selector9/1 -> Derivative3/1, Bus Creator6/19  "nWheelRR_radps"
  Bus Selector3/1 -> Signal Specification1/1  "<phi_IK_rad>"
  Add/1 -> Bus Creator6/6  "psi_rad"
  Bus Selector5/1 -> Signal Specification2/1  "<v_K_IK_mps>"
  Matrix Multiply1/1 -> Selector5/1, Selector3/1, Selector4/1
  Selector6/1 -> Derivative/1, Bus Creator6/16  "nWheelFL_radps"
  SimDualTrackModel/1 -> Bus Selector2/1, Bus Selector/1, Bus Selector1/1, Bus Selector5/1, Bus Selector3/1, Bus Selector4/1
  Bus Selector1/1 -> Signal Specification3/1  "<omega_K_IK_radps>"
  Matrix Multiply4/1 -> Selector15/1, Selector13/1, Selector14/1
  Matrix Multiply3/1 -> Selector12/1, Selector10/1, Selector11/1
  Selector7/1 -> Derivative1/1, Bus Creator6/17  "nWheelFR_radps"
  A_down_up/1 -> Matrix Multiply4/1, Matrix Multiply/1, Matrix Multiply1/1, Matrix Multiply2/1, Matrix Multiply3/1
  Selector10/1 -> Bus Creator6/4  "phi_rad"
  Selector15/1 -> Bus Creator6/3  "z_m"
  Selector8/1 -> Derivative2/1, Bus Creator6/18  "nWheelRL_radps"
  Bus Selector/1 -> Signal Specification4/1  "<a_K_IK_mps2>"
  Selector13/1 -> Bus Creator6/1  "x_m"
  Selector5/1 -> Bus Creator6/12  "dPsi_radps"
  Selector/1 -> Bus Creator6/13  "ax_mps2"
  Signal Specification/1 -> Matrix Multiply4/2
  Signal Specification1/1 -> Matrix Multiply3/2
  Signal Specification2/1 -> Matrix Multiply2/2
  Signal Specification3/1 -> Matrix Multiply1/2
  Signal Specification4/1 -> Matrix Multiply/2
  Signal Specification5/1 -> Selector9/1, Selector8/1, Selector7/1, Selector6/1
  Selector11/1 -> Bus Creator6/5  "theta_rad"
  Selector18/1 -> Bus Creator6/9  "vz_mps"
  Selector3/1 -> Bus Creator6/10  "dPhi_radps"
  Selector4/1 -> Bus Creator6/11  "dTheta_radps"
  Selector2/1 -> Bus Creator6/15  "az_mps2"
  Bus Creator6/1 -> SimRealState/1
  Constant/1 -> Add/2
  Selector12/1 -> Add/1
  SteeringAngle/1 -> Signal Conversion/1
  Signal Conversion/1 -> Bus Creator6/20  "DeltaWheel_rad"
  Derivative/1 -> Bus Creator6/21  "dnWheelFL_radps2"
  Derivative1/1 -> Bus Creator6/22  "dnWheelFR_radps2"
  Derivative2/1 -> Bus Creator6/23  "dnWheelRL_radps2"
  Derivative3/1 -> Bus Creator6/24  "dnWheelRR_radps2"
